simulink model "lin_3dof_surface_vessel_model_1_2021"  (R2021b)
settings: Solver=VariableStepAuto  StartTime=0.0  StopTime=50
InitFcn:
  | % Rigid body
  | m = 127.92;
  | I_z = 61.967;
  | x_g = 0;
  | 
  | % Added mass
  | X_du = 3.262;
  | Y_dv = 28.89;
  | Y_dr = 0.525;
  | N_dv = 0.157;
  | N_dr = 13.98;
  | 
  | % Linear drag coefficients
  | X_u = -2.332;
  | Y_v = -4.673;
  | N_r = -0.01675;
  | Y_r = 0;
  | N_v = 0;
  | 
  | M = [m-X_du 0 0;
  |     0 m-Y_dv m*x_g-Y_dr;
  |     0 m*x_g-Y_dr I_z-N_dr];
  | 
  | D = [X_u 0 0;
  |     0 Y_v Y_r;
  |     0 N_v N_r];
  | 
  | eta_0 = [0.8; 0.2; 0];
values from neighbouring files (symbols this model uses):
  A_0 = [-kappa.*C_2 eye(3); -kappa.*kappa.*C_1 zeros(3,3)]    [initialization.m]
  B_0 = kappa.*[C_2; kappa.*C_1]    [initialization.m]
  initial = x.data(:, 1, 1)    [initialization.m]
  K = [25 0 0 100 0 0; 0 75 0 0 100 0; 0 0 1000 0 0 100]    [initialization.m]
  Kdy = 100    [coeffs.m]
  Kiphi = 1    [coeffs.m]
  Kix = 1    [coeffs.m]
  Kiy = 1    [coeffs.m]
  Kpphi = 200    [coeffs.m]
  Kpx = 30    [coeffs.m]
  Kpy = 20    [coeffs.m]
  lambda = 10    [initialization.m]
libraries: slpidlib x3
settings Model: Creator=olegborisov  LastModifiedBy=kirba
settings SolverCC: AlgebraicLoopSolver=TrustRegion
settings DataIOCC: ReturnWorkspaceOutputs=off

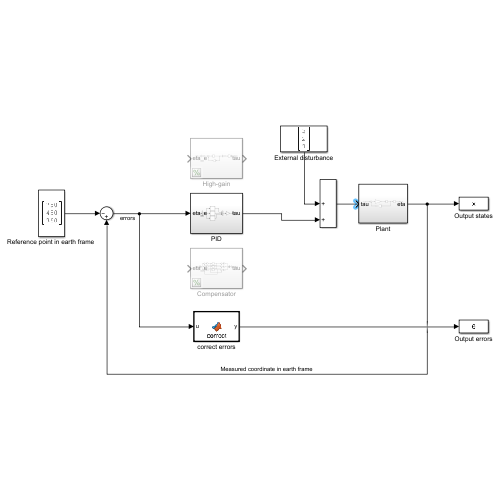
[thumbnail: Simulink's stored preview of the top-level diagram]
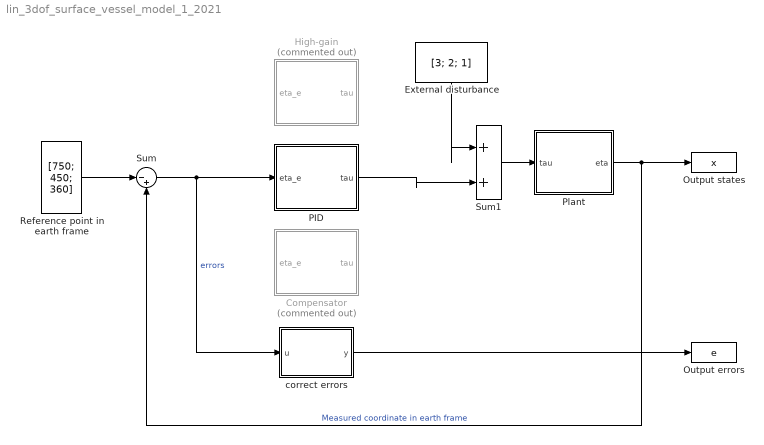
== system lin_3dof_surface_vessel_model_1_2021 ==
  Compensator : Subsystem  Commented=on
  External disturbance : Constant  Value=[3; 2; 1]  VectorParams1D=off
  High-gain : Subsystem  Commented=on
  Output errors : ToWorkspace  VariableName=e  SaveFormat=Timeseries  SampleTime=-1
  Output states : ToWorkspace  VariableName=x  SaveFormat=Timeseries  SampleTime=-1
  PID : Subsystem
  Plant : Subsystem
  "Reference point in earth frame " : Constant  Value=[750; 450; 360]  VectorParams1D=off
  Sum : Sum  Inputs=|-+
  Sum1 : Sum  Inputs=|++
  correct errors : MATLAB Function  TreatAsAtomicUnit=on
  wires:
  Plant/1(eta) -> Sum/2, Output states/1  "Measured coordinate in earth frame"
  "Reference point in earth frame "/1 -> Sum/1
  Sum/1 -> PID/1(eta_e), correct errors/1(u)  "errors"
  correct errors/1(y) -> Output errors/1
  External disturbance/1 -> Sum1/1
  Sum1/1 -> Plant/1(tau)
  PID/1(tau) -> Sum1/2

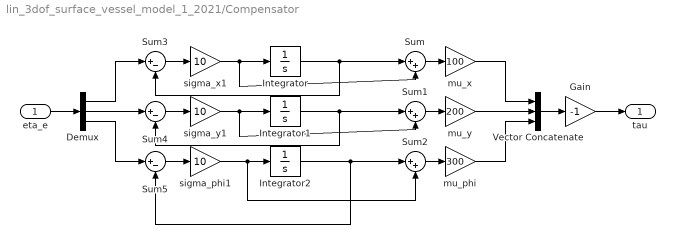
== system lin_3dof_surface_vessel_model_1_2021/Compensator ==
  eta_e : Inport
  Demux : Demux  Outputs=3
  Gain : Gain  Gain=-1
  Integrator : Integrator
  Integrator1 : Integrator
  Integrator2 : Integrator
  Sum : Sum  Inputs=|++
  Sum1 : Sum  Inputs=|++
  Sum2 : Sum  Inputs=|++
  Sum3 : Sum  Inputs=|+-
  Sum4 : Sum  Inputs=|+-
  Sum5 : Sum  Inputs=|+-
  Vector Concatenate : Concatenate  NumInputs=3
  mu_phi : Gain  Gain=300
  mu_x : Gain  Gain=100
  mu_y : Gain  Gain=200
  sigma_phi1 : Gain  Gain=10
  sigma_x1 : Gain  Gain=10
  sigma_y1 : Gain  Gain=10
  tau : Outport
  wires:
  Vector Concatenate/1 -> Gain/1
  eta_e/1 -> Demux/1
  Demux/1 -> Sum3/1
  Demux/2 -> Sum4/1
  Demux/3 -> Sum5/1
  mu_x/1 -> Vector Concatenate/1
  mu_y/1 -> Vector Concatenate/2
  mu_phi/1 -> Vector Concatenate/3
  Gain/1 -> tau/1
  Sum/1 -> mu_x/1
  Sum1/1 -> mu_y/1
  Sum2/1 -> mu_phi/1
  Integrator/1 -> Sum3/2, Sum/1
  Integrator1/1 -> Sum4/2, Sum1/1
  Integrator2/1 -> Sum5/2, Sum2/1
  Sum3/1 -> sigma_x1/1
  Sum4/1 -> sigma_y1/1
  Sum5/1 -> sigma_phi1/1
  sigma_x1/1 -> Sum/2, Integrator/1
  sigma_y1/1 -> Sum1/2, Integrator1/1
  sigma_phi1/1 -> Sum2/2, Integrator2/1

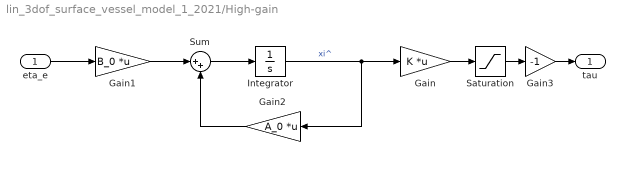
== system lin_3dof_surface_vessel_model_1_2021/High-gain ==
  eta_e : Inport
  Gain : Gain  Gain=K  Multiplication=Matrix(K*u)
  Gain1 : Gain  Gain=B_0  Multiplication=Matrix(K*u)
  Gain2 : Gain  Gain=A_0  Multiplication=Matrix(K*u)
  Gain3 : Gain  Gain=-1
  Integrator : Integrator
  Saturation : Saturate  UpperLimit=lambda  LowerLimit=-lambda
  Sum : Sum  Inputs=|++
  tau : Outport
  wires:
  Integrator/1 -> Gain/1, Gain2/1  "xi^"
  Gain/1 -> Saturation/1
  Saturation/1 -> Gain3/1
  Gain1/1 -> Sum/1
  Gain2/1 -> Sum/2
  Sum/1 -> Integrator/1
  eta_e/1 -> Gain1/1
  Gain3/1 -> tau/1

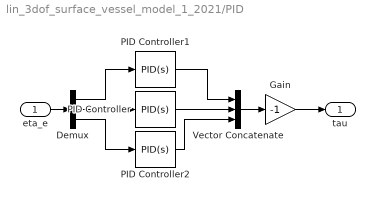
== system lin_3dof_surface_vessel_model_1_2021/PID ==
  eta_e : Inport
  Demux : Demux  Outputs=3
  Gain : Gain  Gain=-1
  PID Controller : slpidlib/PID Controller  Controller=PID  Form=Parallel  TimeDomain=Continuous-time  UseExternalTs=off  SampleTime=-1  IntegratorMethod=Forward Euler  FilterMethod=Forward Euler  ControllerParametersSource=internal  P=Kpy  I=Kiy  D=Kdy  UseFilter=on  N=100  TunerSelectOption=Transfer Function Based (PID Tuner App)  InitialConditionSource=internal  InitialConditionForIntegrator=0  InitialConditionForFilter=0  DifferentiatorICPrevScaledInput=0  ExternalReset=none  TrackingMode=off  Kt=1  LimitOutput=off  SatLimitsSource=internal  UpperSaturationLimit=inf  LowerSaturationLimit=-inf  LinearizeAsGain=on  AntiWindupMode=none  Kb=1  POutMin=[]  POutMax=[]  IOutMin=[]  IOutMax=[]  DOutMin=[]  DOutMax=[]  NOutMin=[]  NOutMax=[]  SumOutMin=[]  SumOutMax=[]  SaturationOutMin=[]  SaturationOutMax=[]  PParamMin=[]  PParamMax=[]  IParamMin=[]  IParamMax=[]  DParamMin=[]  DParamMax=[]  NParamMin=[]  NParamMax=[]  KbParamMin=[]  KbParamMax=[]  KtParamMin=[]  KtParamMax=[]  KbOutMin=[]  KbOutMax=[]  KtOutMin=[]  KtOutMax=[]  IntegratorOutMin=[]  IntegratorOutMax=[]  FilterOutMin=[]  FilterOutMax=[]  SumI1OutMin=[]  SumI1OutMax=[]  SumI2OutMin=[]  SumI2OutMax=[]  SumI3OutMin=[]  SumI3OutMax=[]  SumI4OutMin=[]  SumI4OutMax=[]  SumDOutMin=[]  SumDOutMax=[]  DifferentiatorOutMin=[]  DifferentiatorOutMax=[]  FilterDiffOutCoefMin=[]  FilterDiffOutCoefMax=[]  ReciprocalOutMin=[]  ReciprocalOutMax=[]  SumDenOutMin=[]  SumDenOutMax=[]  SumNumOutMin=[]  SumNumOutMax=[]  DivideOutMin=[]  DivideOutMax=[]  UdiffTsProdOutMin=[]  UdiffTsProdOutMax=[]  NTsProdOutMin=[]  NTsProdOutMax=[]  UintegralTsProdOutMin=[]  UintegralTsProdOutMax=[]  UngainTsProdOutMin=[]  UngainTsProdOutMax=[]  IntegratorContinuousStateAttributes=''  IntegratorStateMustResolveToSignalObject=off  IntegratorRTWStateStorageClass=Auto  FilterContinuousStateAttributes=''  FilterStateMustResolveToSignalObject=off  FilterRTWStateStorageClass=Auto  ParallelPVariant=InternalParameters  IdealPVariant=Disabled  IVariant=InternalParameters  DVariant=InternalParameters  IntegratorVariant=Continuous  SatVariant=Disabled  AWVariant=Passthrough  PCopyVariant=Disabled  TRVariant=Disabled  FdbkBlocksVariant=Forward  IdealPFdbkVariant=Disabled  SatFdbkVariant=Disabled  DerivativeFilterVariant=ContFilter  NVariant=InternalParameters  NCopyVariant=Disabled  FilterICVariant=InternalICsFilter  IntegratorICVariant=InternalICs  ExternalResetVariant=Disabled  TRSumVariant=Passthrough  SumFdbkVariant=Disabled  SumVariant=Sum_PID  TsampFilterVariant=InternalTs  TsampNgainVariant=Passthrough  TsampIntegralVariant=Passthrough  ExternalSaturationOutDataTypeStr=Inherit: Same as second input
  PID Controller1 : slpidlib/PID Controller  Controller=PID  Form=Parallel  TimeDomain=Continuous-time  UseExternalTs=off  SampleTime=-1  IntegratorMethod=Forward Euler  FilterMethod=Forward Euler  ControllerParametersSource=internal  P=Kpx  I=Kix  D=Kpx  UseFilter=on  N=100  TunerSelectOption=Frequency Response Based  InitialConditionSource=internal  InitialConditionForIntegrator=0  InitialConditionForFilter=0  DifferentiatorICPrevScaledInput=0  ExternalReset=none  TrackingMode=off  Kt=1  LimitOutput=off  SatLimitsSource=internal  UpperSaturationLimit=inf  LowerSaturationLimit=-inf  LinearizeAsGain=on  AntiWindupMode=none  Kb=1  POutMin=[]  POutMax=[]  IOutMin=[]  IOutMax=[]  DOutMin=[]  DOutMax=[]  NOutMin=[]  NOutMax=[]  SumOutMin=[]  SumOutMax=[]  SaturationOutMin=[]  SaturationOutMax=[]  PParamMin=[]  PParamMax=[]  IParamMin=[]  IParamMax=[]  DParamMin=[]  DParamMax=[]  NParamMin=[]  NParamMax=[]  KbParamMin=[]  KbParamMax=[]  KtParamMin=[]  KtParamMax=[]  KbOutMin=[]  KbOutMax=[]  KtOutMin=[]  KtOutMax=[]  IntegratorOutMin=[]  IntegratorOutMax=[]  FilterOutMin=[]  FilterOutMax=[]  SumI1OutMin=[]  SumI1OutMax=[]  SumI2OutMin=[]  SumI2OutMax=[]  SumI3OutMin=[]  SumI3OutMax=[]  SumI4OutMin=[]  SumI4OutMax=[]  SumDOutMin=[]  SumDOutMax=[]  DifferentiatorOutMin=[]  DifferentiatorOutMax=[]  FilterDiffOutCoefMin=[]  FilterDiffOutCoefMax=[]  ReciprocalOutMin=[]  ReciprocalOutMax=[]  SumDenOutMin=[]  SumDenOutMax=[]  SumNumOutMin=[]  SumNumOutMax=[]  DivideOutMin=[]  DivideOutMax=[]  UdiffTsProdOutMin=[]  UdiffTsProdOutMax=[]  NTsProdOutMin=[]  NTsProdOutMax=[]  UintegralTsProdOutMin=[]  UintegralTsProdOutMax=[]  UngainTsProdOutMin=[]  UngainTsProdOutMax=[]  IntegratorContinuousStateAttributes=''  IntegratorStateMustResolveToSignalObject=off  IntegratorRTWStateStorageClass=Auto  FilterContinuousStateAttributes=''  FilterStateMustResolveToSignalObject=off  FilterRTWStateStorageClass=Auto  ParallelPVariant=InternalParameters  IdealPVariant=Disabled  IVariant=InternalParameters  DVariant=InternalParameters  IntegratorVariant=Continuous  SatVariant=Disabled  AWVariant=Passthrough  PCopyVariant=Disabled  TRVariant=Disabled  FdbkBlocksVariant=Forward  IdealPFdbkVariant=Disabled  SatFdbkVariant=Disabled  DerivativeFilterVariant=ContFilter  NVariant=InternalParameters  NCopyVariant=Disabled  FilterICVariant=InternalICsFilter  IntegratorICVariant=InternalICs  ExternalResetVariant=Disabled  TRSumVariant=Passthrough  SumFdbkVariant=Disabled  SumVariant=Sum_PID  TsampFilterVariant=InternalTs  TsampNgainVariant=Passthrough  TsampIntegralVariant=Passthrough  ExternalSaturationOutDataTypeStr=Inherit: Same as second input
  PID Controller2 : slpidlib/PID Controller  Controller=PID  Form=Parallel  TimeDomain=Continuous-time  UseExternalTs=off  SampleTime=-1  IntegratorMethod=Forward Euler  FilterMethod=Forward Euler  ControllerParametersSource=internal  P=Kpphi  I=Kiphi  D=Kpphi  UseFilter=on  N=100  TunerSelectOption=Transfer Function Based (PID Tuner App)  InitialConditionSource=internal  InitialConditionForIntegrator=0  InitialConditionForFilter=0  DifferentiatorICPrevScaledInput=0  ExternalReset=none  TrackingMode=off  Kt=1  LimitOutput=off  SatLimitsSource=internal  UpperSaturationLimit=inf  LowerSaturationLimit=-inf  LinearizeAsGain=on  AntiWindupMode=none  Kb=1  POutMin=[]  POutMax=[]  IOutMin=[]  IOutMax=[]  DOutMin=[]  DOutMax=[]  NOutMin=[]  NOutMax=[]  SumOutMin=[]  SumOutMax=[]  SaturationOutMin=[]  SaturationOutMax=[]  PParamMin=[]  PParamMax=[]  IParamMin=[]  IParamMax=[]  DParamMin=[]  DParamMax=[]  NParamMin=[]  NParamMax=[]  KbParamMin=[]  KbParamMax=[]  KtParamMin=[]  KtParamMax=[]  KbOutMin=[]  KbOutMax=[]  KtOutMin=[]  KtOutMax=[]  IntegratorOutMin=[]  IntegratorOutMax=[]  FilterOutMin=[]  FilterOutMax=[]  SumI1OutMin=[]  SumI1OutMax=[]  SumI2OutMin=[]  SumI2OutMax=[]  SumI3OutMin=[]  SumI3OutMax=[]  SumI4OutMin=[]  SumI4OutMax=[]  SumDOutMin=[]  SumDOutMax=[]  DifferentiatorOutMin=[]  DifferentiatorOutMax=[]  FilterDiffOutCoefMin=[]  FilterDiffOutCoefMax=[]  ReciprocalOutMin=[]  ReciprocalOutMax=[]  SumDenOutMin=[]  SumDenOutMax=[]  SumNumOutMin=[]  SumNumOutMax=[]  DivideOutMin=[]  DivideOutMax=[]  UdiffTsProdOutMin=[]  UdiffTsProdOutMax=[]  NTsProdOutMin=[]  NTsProdOutMax=[]  UintegralTsProdOutMin=[]  UintegralTsProdOutMax=[]  UngainTsProdOutMin=[]  UngainTsProdOutMax=[]  IntegratorContinuousStateAttributes=''  IntegratorStateMustResolveToSignalObject=off  IntegratorRTWStateStorageClass=Auto  FilterContinuousStateAttributes=''  FilterStateMustResolveToSignalObject=off  FilterRTWStateStorageClass=Auto  ParallelPVariant=InternalParameters  IdealPVariant=Disabled  IVariant=InternalParameters  DVariant=InternalParameters  IntegratorVariant=Continuous  SatVariant=Disabled  AWVariant=Passthrough  PCopyVariant=Disabled  TRVariant=Disabled  FdbkBlocksVariant=Forward  IdealPFdbkVariant=Disabled  SatFdbkVariant=Disabled  DerivativeFilterVariant=ContFilter  NVariant=InternalParameters  NCopyVariant=Disabled  FilterICVariant=InternalICsFilter  IntegratorICVariant=InternalICs  ExternalResetVariant=Disabled  TRSumVariant=Passthrough  SumFdbkVariant=Disabled  SumVariant=Sum_PID  TsampFilterVariant=InternalTs  TsampNgainVariant=Passthrough  TsampIntegralVariant=Passthrough  ExternalSaturationOutDataTypeStr=Inherit: Same as second input
  Vector Concatenate : Concatenate  NumInputs=3
  tau : Outport
  wires:
  Vector Concatenate/1 -> Gain/1
  eta_e/1 -> Demux/1
  Demux/1 -> PID Controller1/1
  Demux/2 -> PID Controller/1
  Demux/3 -> PID Controller2/1
  PID Controller1/1 -> Vector Concatenate/1
  PID Controller/1 -> Vector Concatenate/2
  PID Controller2/1 -> Vector Concatenate/3
  Gain/1 -> tau/1

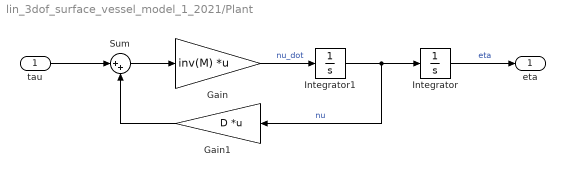
== system lin_3dof_surface_vessel_model_1_2021/Plant ==
  tau : Inport
  Gain : Gain  Gain=inv(M)  Multiplication=Matrix(K*u) (u vector)
  Gain1 : Gain  Gain=D  Multiplication=Matrix(K*u) (u vector)
  Integrator : Integrator  InitialCondition=initial
  Integrator1 : Integrator
  Sum : Sum  Inputs=|++
  eta : Outport
  wires:
  Integrator1/1 -> Integrator/1, Gain1/1  "nu"
  Gain/1 -> Integrator1/1  "nu_dot"
  Sum/1 -> Gain/1
  tau/1 -> Sum/1
  Gain1/1 -> Sum/2
  Integrator/1 -> eta/1  "eta"

== matlab function lin_3dof_surface_vessel_model_1_2021/correct errors ==
  data: u input; y output
function y = correct(u)

q = [1 0 0;
    0 -1 0;
    0 0 -1];

y = q*u;
